simulink model "Test_ParamModel"  (R2020a)
settings: Solver=FixedStepAuto  StartTime=0.0  StopTime=10.0  FixedStep=0.1  MaxStep=0.1  RelTol=1e-3
model workspace (MAT data in the model file):
  param1 = Simulink.Parameter
  param1.Value = 1
  param1.DataType = 'double'
  param1.Dimensions = [1 1]
  param2 = Simulink.Parameter
  param2.Value = -1
  param2.DataType = 'int8'
  param2.Dimensions = [1 1]
  unusedParam = Simulink.Parameter
  unusedParam.Value = 4
  unusedParam.DataType = 'auto'
  unusedParam.Dimensions = [1 1]
values from neighbouring files (symbols this model uses):
  param3 = 3.0    [ParamDD.sldd]
settings Model: DataDictionary=ParamDD.sldd  OrderedModelArguments=off  Creator=tomha  LastModifiedBy=toma
settings OptimizationCC: DefaultParameterBehavior=Inlined  EnhancedBackFolding=on  PassReuseOutputArgsAs=Individual arguments  ZeroExternalMemoryAtStartup=off  ZeroInternalMemoryAtStartup=off  OptimizeBlockOrder=speed  DifferentSizesBufferReuse=on  OptimizationCustomize=off  EfficientTunableParamExpr=on
settings DebuggingCC: UnderspecifiedInitializationDetection=Classic  MergeDetectMultiDrivingBlocksExec=none  ParameterTunabilityLossMsg=error  ModelReferenceSymbolNameMessage=none
settings ModelReferenceCC: PropagateSignalLabelsOutOfModel=off
settings SFSimCC: MATLABDynamicMemAlloc=off
settings RTWCC: Description=CIGRE export target  SystemTargetFile=cigre.tlc  TemplateMakefile=cigre_tmf  Toolchain=CIGRE DLL - Microsoft Visual C++ 2019 (64bit) | nmake makefile (64-bit Windows)
settings CodeAppCC: ForceParamTrailComments=on  IgnoreCustomStorageClasses=off  OperatorAnnotations=on  SimulinkDataObjDesc=on  SFDataObjDesc=on  InsertBlockDesc=on
settings STFCustomTargetCC: TargetLangStandard=C99 (ISO)  MultiwordLength=256  GenerateSampleERTMain=on  CompOptLevelCompliant=on  CombineOutputUpdateFcns=on  ERTCustomFileBanners=on  MultiInstanceERTCode=on  CodeInterfacePackaging=Reusable function  SupportContinuousTime=off  SupportNonInlinedSFcns=off  RemoveResetFunc=on  MATLABClassNameForMDSCustomization=Simulink.SoftwareTarget.ERTCustomization  UseToolchainInfoCompliant=on  SystemTargetFile=cigre.tlc
settings ERTTargetCC: TargetLangStandard=C99 (ISO)  GenerateSampleERTMain=on  ParMdlRefBuildCompliant=off  ConcurrentExecutionCompliant=off  MultiInstanceERTCode=on  CodeInterfacePackaging=Reusable function  ModelStepFunctionPrototypeControlCompliant=off  CPPClassGenCompliant=off  InlinedParameterPlacement=NonHierarchical  RootIOFormat=Structure reference  ERTCustomFileTemplate=example_file_process.tlc

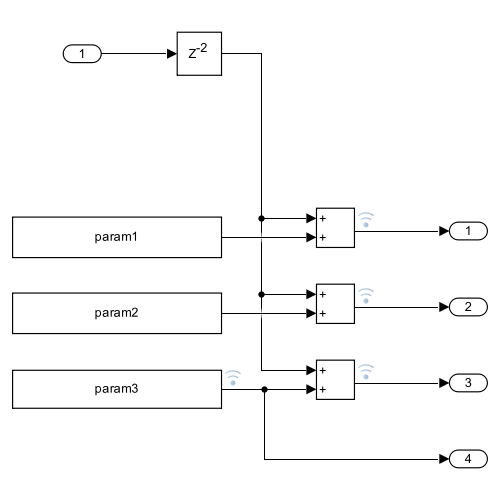
[thumbnail: Simulink's stored preview of the top-level diagram]
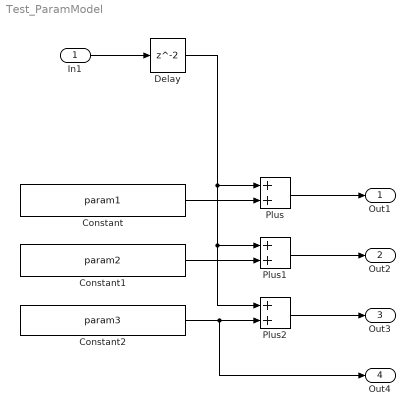
== system Test_ParamModel ==
  In1 : Inport
  Constant : Constant  Value=param1
  Constant1 : Constant  Value=param2
  Constant2 : Constant  Value=param3
  Delay : Delay
  Plus : Sum
  Plus1 : Sum
  Plus2 : Sum
  Out1 : Outport
  Out2 : Outport  Port=2
  Out3 : Outport  Port=3
  Out4 : Outport  Port=4
  wires:
  Constant/1 -> Plus/2
  In1/1 -> Delay/1
  Plus/1 -> Out1/1
  Delay/1 -> Plus1/1, Plus2/1, Plus/1
  Constant1/1 -> Plus1/2
  Plus1/1 -> Out2/1
  Plus2/1 -> Out3/1
  Constant2/1 -> Out4/1, Plus2/2
